simulink model "Eq_1"  (R2014a)
settings: Solver=ode45  StartTime=0.0  StopTime=20  RelTol=1e-3
undefined symbols (not defined in the file or in its folder): dfilt
libraries: dsparch4 x5, dspvision x2, dspsnks4 x1
settings Model: Creator=Misa  LastModifiedBy=Misa

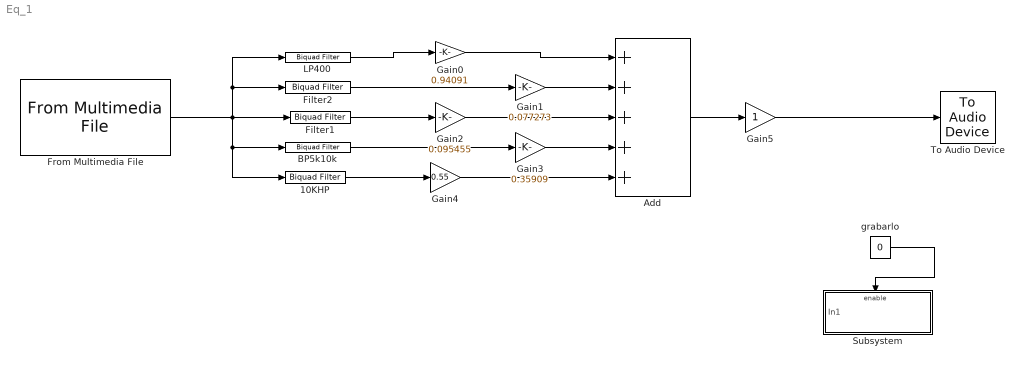
== system Eq_1 ==
  10KHP : dsparch4/Biquad Filter  Tag=BlockMethodSubSystem  IIRFiltStruct=Direct form II  CoeffSource=Specify via dialog  BiQuadCoeffs=[1 -2 1 1 -0.435559960227692333 0.682874457925469414;1 -2 1 1 -0.336863684852461154 0.301541332551575114;1 -2 1 1 -0.287076251600125121 0.109177462139277051;1 -2 1 1 -0.265814507780955722 0.0270283922717663959]  a0Flag=Warning  IC=0  ICnum=0  ICden=0  InputProcessing=Columns as channels (frame based)  denAccumFracLength=30  denProdOutputFracLength=30  secondMemoryFracLength=15  roundingMode=Floor  overflowMode=off  ScaleValues=[0.529608604538290506;0.409601254351009081;0.349063428434850553;0.323210725013180544;1]  optimizeScaleValues=on  ScaleValueMode=Specify via input port (g)  scaleValueFracLength=14  FilterSource=Specify via dialog  dfiltObjectName=dfilt.df2tsos([1 0.3 0.4],[1 0.1 0.2])
  Add : Sum  Inputs=+++++
  BP5k10k : dsparch4/Biquad Filter  Tag=BlockMethodSubSystem  IIRFiltStruct=Direct form II  CoeffSource=Specify via dialog  BiQuadCoeffs=[1 0 -1 1 -0.511936060109229096 0.976812733722258741;1 0 -1 1 -1.5749417552576479 0.98532114132335924;1 0 -1 1 -1.55120780296343908 0.956591366841473167;1 0 -1 1 -0.5026942036248776 0.932090235078945284;1 0 -1 1 -0.496206083464974634 0.889564263737497196;1 0 -1 1 -1.52719342803245395 0.928655042129086672;1 0 -1 1 -1.50288428756205406 0.901464029452747728;1 0 -1 1 -0.492327906370097379 0.849219797568050661;1 0 -1 1 -1.47826174218308015 0.874975513981652409;1 0 -1 1 -0.490928978268946159 0.811036332045524389;1 0 -1 1 -1.45330358333625353 0.849152306076616625;1 0 -1 1 -0.491891608264251601 0.774990857026918945;1 0 -1 1 -1.42798470855204052 0.823963188122787571;1 0 -1 1 -0.495110695998242645 0.741060291658979464;1 0 -1 1 -1.40227778727378527 0.799383332368227784;1 0 -1 1 -0.500493064212129246 0.70922346320206564;1 0 -1 1 -1.37615396097244957 0.775394812461079219;1 0 -1 1 -0.507956573002034784 0.679462697186595799;1 0 -1 1 -1.34958362384959907 0.7519872274617736;1 0 -1 1 -0.517429030514883981 0.651765066895615197;1 0 -1 1 -1.32253733382701011 0.72915845201805296;1 0 -1 1 -0.528846896304387082 0.626123329774780357;1 0 -1 1 -1.29498690690488116 0.706915518856455316;1 0 -1 1 -0.542153758407436959 0.602536556936418166;1 0 -1 1 -1.26690674987356156 0.685275628197983599;1 0 -1 1 -0.557298554215037045 0.581010439505093901;1 0 -1 1 -1.23827548448857305 0.664267261325699687;1 0 -1 1 -0.574233500145569953 0.561557232705398368;1 0 -1 1 -1.20907790720441133 0.643931350446522721;1 0 -1 1 -0.592911698886189553 0.544195276865696909;1 0 -1 1 -1.17930730791784777 0.624322422786211417;1 0 -1 1 -0.613284409671686737 0.528948017042816243;1 0 -1 1 -1.14896813361933203 0.605509593538764546;1 0 -1 1 -0.635298001700298487 0.515842435093875618;1 0 -1 1 -1.11807892346795779 0.587577232772038549;1 0 -1 1 -0.658890668031314686 0.504906817560012877;1 0 -1 1 -1.08667535838030926 0.570625083388540011;1 0 -1 1 -0.683989059197508409 0.496167819434113699;1 0 -1 1 -1.05481316500134237 0.5547675749297305;1 0 -1 1 -0.710505097907362604 0.489646857192791884;1 0 -1 1 -1.02257050610441946 0.540132082055159723;1 0 -1 1 -0.738333343299314659 0.485355978860020243;1 0 -1 1 -0.990049406305708146 0.526855940429187597;1 0 -1 1 -0.767349355898213625 0.483293507046987036;1 0 -1 1 -0.957375744728905631 0.515082173873032012;1 0 -1 1 -0.797409531394399407 0.483439907073740183;1 0 -1 1 -0.924697436908860082 0.504954102663914828;1 0 -1 1 -0.828352780577823244 0.485754450371230106;1 0 -1 1 -0.892180648569675938 0.49660925926267574;1 0 -1 1 -0.860004212382262767 0.490173266415208975]  a0Flag=Warning  IC=0  ICnum=0  ICden=0  InputProcessing=Columns as channels (frame based)  denAccumFracLength=30  denProdOutputFracLength=30  secondMemoryFracLength=15  roundingMode=Floor  overflowMode=off  ScaleValues=[0.318409620604874377;0.318409620604874377;0.312609545517313181;0.312609545517313181;0.307147001457118485;0.307147001457118485;0.302011246073271178;0.302011246073271178;0.29719133618218585;0.29719133618218585;0.292676349944423264;0.292676349944423264;0.288455556702515381;0.288455556702515381;0.284518544849641064;0.284518544849641064;0.280855316314686354;0.280855316314686354;0.277456354711022701;0.277456354711022701;0.274312672892673248;0.274312672892673248;0.271415844571001152;0.271415844571001152;0.268758023742088736;0.268758023742088736;0.266331954933413495;0.266331954933413495;0.264130976673456697;0.264130976673456697;0.262149020097042551;0.262149020097042551;0.260380604202797961;0.260380604202797961;0.258820828960209026;0.258820828960209026;0.257465367207995455;0.257465367207995455;0.2563104560809355;0.2563104560809355;0.255352888538870559;0.255352888538870559;0.254590005441150902;0.254590005441150902;0.254019688505433716;0.254019688505433716;0.253640354405854029;0.253640354405854029;0.253450950197460445;0.253450950197460445;1]  optimizeScaleValues=on  ScaleValueMode=Specify via input port (g)  scaleValueFracLength=14  FilterSource=Specify via dialog  dfiltObjectName=dfilt.df2tsos([1 0.3 0.4],[1 0.1 0.2])
  Filter1 : dsparch4/Biquad Filter  Tag=BlockMethodSubSystem  IIRFiltStruct=Direct form II  CoeffSource=Specify via dialog  BiQuadCoeffs=[1 0 -1 1 -1.49298544457669613 0.972536600913176619;1 0 -1 1 -1.97375600080993996 0.993967196611222681;1 0 -1 1 -1.45434811513615525 0.91992215302516156;1 0 -1 1 -1.96184279045341059 0.981990541850511933;1 0 -1 1 -1.41911007136003064 0.870355402822089896;1 0 -1 1 -1.94995566918991003 0.970098550984774155;1 0 -1 1 -1.38714659148742636 0.823781823951208914;1 0 -1 1 -1.93805449177893774 0.958251256010940966;1 0 -1 1 -1.35833576516020438 0.780137916222685357;1 0 -1 1 -1.92609852985326024 0.946408948977047637;1 0 -1 1 -1.33256154535689264 0.739355628990374436;1 0 -1 1 -1.91404574389860604 0.934531500155876826;1 0 -1 1 -1.3097162226504544 0.701366035921648701;1 0 -1 1 -1.90185198328248095 0.922577639450826381;1 0 -1 1 -1.28970250064079539 0.666102437361354771;1 0 -1 1 -1.88947007254741828 0.910504166064626363;1 0 -1 1 -1.27243533948969301 0.633503055805215709;1 0 -1 1 -1.87684873043618161 0.898265043581852884;1 0 -1 1 -1.86393124983616087 0.885810324816448391;1 0 -1 1 -1.257843732058602 0.603513485803715;1 0 -1 1 -1.85065383861322852 0.8730848306789043;1 0 -1 1 -1.24587258765892894 0.576089065158300606;1 0 -1 1 -1.83694347738664909 0.860026475874825724;1 0 -1 1 -1.23648492746493122 0.551197354350352553;1 0 -1 1 -1.82271508070995703 0.846564084478204637;1 0 -1 1 -1.22966465290023219 0.528820953727261345;1 0 -1 1 -1.8078676351395444 0.832614457983713696;1 0 -1 1 -1.22542025119886655 0.508960967165100642;1 0 -1 1 -1.79227879867224105 0.81807832481258369;1 0 -1 1 -1.22378998315903997 0.491641562843065538;1 0 -1 1 -1.77579711858101463 0.802834570778408141;1 0 -1 1 -1.22484941898211241 0.476916336802188867;1 0 -1 1 -1.75823043384986621 0.786731740493668341;1 0 -1 1 -1.22872277367223726 0.464877654925497041;1 0 -1 1 -1.73932791135376363 0.769575035828907961;1 0 -1 1 -1.23560060637514946 0.455671050426820101;1 0 -1 1 -1.71875093669712986 0.751105539894514784;1 0 -1 1 -1.24576867300432736 0.449518575540772625;1 0 -1 1 -1.69602335791846537 0.730965293920004311;1 0 -1 1 -1.25965744166257498 0.44675892609350043;1 0 -1 1 -1.67044089099015647 0.708635073665359383;1 0 -1 1 -1.27793246767386881 0.447921223551549119;1 0 -1 1 -1.64089382056394095 0.683316374884235245;1 0 -1 1 -1.30167149900252088 0.453871915193899855;1 0 -1 1 -1.60549565687988194 0.653697459997890973;1 0 -1 1 -1.33273565421145501 0.466132696577705508;1 0 -1 1 -1.56082757662151606 0.617543327540308828;1 0 -1 1 -1.3745248473673557 0.487583520094362788;1 0 -1 1 -1.50169156008034421 0.572103291046450191;1 0 -1 1 -1.43222454905332985 0.523165952149703961]  a0Flag=Warning  IC=0  ICnum=0  ICden=0  InputProcessing=Columns as channels (frame based)  denAccumFracLength=30  denProdOutputFracLength=30  secondMemoryFracLength=15  roundingMode=Floor  overflowMode=off  ScaleValues=[0.278758877019711249;0.278758877019711249;0.274235010892847242;0.274235010892847242;0.269949416623545435;0.269949416623545435;0.265898272850538464;0.265898272850538464;0.262077096217103789;0.262077096217103789;0.258480952180539514;0.258480952180539514;0.255104627583005894;0.255104627583005894;0.251942770859943821;0.251942770859943821;0.248990005094146261;0.248990005094146261;0.246241018460196665;0.246241018460196665;0.243690635976798381;0.243690635976798381;0.241333875910699935;0.241333875910699935;0.239165993663095183;0.239165993663095183;0.237182515518972181;0.237182515518972181;0.235379264249513637;0.235379264249513637;0.233752378222758433;0.233752378222758433;0.232298325392703398;0.232298325392703398;0.231013913295886053;0.231013913295886053;0.229896295981367682;0.229896295981367682;0.22894297862939092;0.22894297862939092;0.228151820470753719;0.228151820470753719;0.227521036498562951;0.227521036498562951;0.227049198362456434;0.227049198362456434;0.226735234749033565;0.226735234749033565;0.226578431477934134;0.226578431477934134;1]  optimizeScaleValues=on  ScaleValueMode=Specify via input port (g)  scaleValueFracLength=14  FilterSource=Specify via dialog  dfiltObjectName=dfilt.df2tsos([1 0.3 0.4],[1 0.1 0.2])
  Filter2 : dsparch4/Biquad Filter  Tag=BlockMethodSubSystem  IIRFiltStruct=Direct form II  CoeffSource=Specify via dialog  BiQuadCoeffs=[1 0 -1 1 -1.97596012833583279 0.996179518646341688;1 0 -1 1 -1.99521952400752611 0.99846517290300385;1 0 -1 1 -1.96851859175579458 0.988605912279289512;1 0 -1 1 -1.99214992198348506 0.995399560857654575;1 0 -1 1 -1.96125803930711751 0.981160151075751497;1 0 -1 1 -1.98907166931553103 0.992334325463347544;1 0 -1 1 -1.95422106977926946 0.973886471810042287;1 0 -1 1 -1.98597866945393919 0.989263518702049982;1 0 -1 1 -1.94744837829074435 0.966827443288640342;1 0 -1 1 -1.98286480675969434 0.986181276643283811;1 0 -1 1 -1.94097871703255276 0.960023914274292345;1 0 -1 1 -1.97972395807416657 0.983081835728266129;1 0 -1 1 -1.93484886261720535 0.953514970993309396;1 0 -1 1 -1.97655001571599565 0.979959562422103359;1 0 -1 1 -1.92909358234205852 0.947337896828783887;1 0 -1 1 -1.97333692733050303 0.976809001648254238;1 0 -1 1 -1.92374559023320169 0.941528125333639165;1 0 -1 1 -1.97007875947474664 0.973624950844582338;1 0 -1 1 -1.91883548183865438 0.936119175780525392;1 0 -1 1 -1.96676979377256256 0.970402568314236436;1 0 -1 1 -1.9143916343797609 0.931142558004078413;1 0 -1 1 -1.96340466691835136 0.967137526832149819;1 0 -1 1 -1.91044005607788758 0.926627630350701614;1 0 -1 1 -1.95997856870902565 0.963826226068218328;1 0 -1 1 -1.90700416542813267 0.922601391201267829;1 0 -1 1 -1.95648751545446853 0.960466080136111344;1 0 -1 1 -1.90410447830915297 0.919088181169101071;1 0 -1 1 -1.95292871913744159 0.957055898955894824;1 0 -1 1 -1.90175817912606515 0.916109270630745209;1 0 -1 1 -1.94930107453028612 0.953596383059907016;1 0 -1 1 -1.94560578572206833 0.950090749581463556;1 0 -1 1 -1.89997855308400165 0.913682307011692396;1 0 -1 1 -1.94184714729627905 0.946545499549337643;1 0 -1 1 -1.89877426304988406 0.911820601091401395;1 0 -1 1 -1.93803348047229917 0.942971320297574023;1 0 -1 1 -1.89814846952970728 0.910532244717123462;1 0 -1 1 -1.93417819657065215 0.939384087834612136;1 0 -1 1 -1.89809782037954733 0.909819078328251596;1 0 -1 1 -1.93030091600834464 0.935805889972775251;1 0 -1 1 -1.89861138115352301 0.909675569333436407;1 0 -1 1 -1.9264285118880915 0.932265934195341317;1 0 -1 1 -1.89966963625802165 0.91008772143071337;1 0 -1 1 -1.92259588239113133 0.928801144878157237;1 0 -1 1 -1.90124375605247531 0.911032202623118792;1 0 -1 1 -1.91884620803054484 0.925456215497890478;1 0 -1 1 -1.90329537329813192 0.912475934793618659;1 0 -1 1 -1.91523045088558952 0.922282894079524906;1 0 -1 1 -1.90577711139492223 0.914376398077903385;1 0 -1 1 -1.91180593584687464 0.91933837367792437;1 0 -1 1 -1.90863402403330928 0.916682834119376344]  a0Flag=Warning  IC=0  ICnum=0  ICden=0  InputProcessing=Columns as channels (frame based)  denAccumFracLength=30  denProdOutputFracLength=30  secondMemoryFracLength=15  roundingMode=Floor  overflowMode=off  ScaleValues=[0.0426725602520760042;0.0426725602520760042;0.0425591023286577275;0.0425591023286577275;0.0424472087389355449;0.0424472087389355449;0.0423372884878717506;0.0423372884878717506;0.0422297336523212302;0.0422297336523212302;0.0421249186567085529;0.0421249186567085529;0.0420231997148002578;0.0420231997148002578;0.0419249144219856346;0.0419249144219856346;0.0418303814820186678;0.0418303814820186678;0.0417399005520427413;0.0417399005520427413;0.0416537521898713708;0.0416537521898713708;0.0415721978878865472;0.0415721978878865472;0.0414954801784973223;0.0414954801784973223;0.0414238227968344447;0.0414238227968344447;0.0413574308872055874;0.0413574308872055874;0.0412964912407680282;0.0412964912407680282;0.0412411725528634698;0.0412411725528634698;0.0411916256894802324;0.0411916256894802324;0.0411479839533424943;0.0411479839533424943;0.0411103633411602012;0.0411103633411602012;0.0410788627845955212;0.0410788627845955212;0.0410535643685060389;0.0410535643685060389;0.0410345335210057505;0.0410345335210057505;0.0410218191708421193;0.0410218191708421193;0.041015453868520603;0.041015453868520603;1]  optimizeScaleValues=on  ScaleValueMode=Specify via input port (g)  scaleValueFracLength=14  FilterSource=Specify via dialog  dfiltObjectName=dfilt.df2tsos([1 0.3 0.4],[1 0.1 0.2])
  From Multimedia File : dspvision/From Multimedia File  inputFilename=/Volumes/DANIEL N/DSP 2016/Calvin Harris - Feel so Close (Original Mix).mp3  loop=on  numPlays=inf  outputStreams=Audio only  videoDataType=single  audioDataType=double  inheritSampleTime=on  userDefinedSampleTime=1/30  noAudioOutput=off  isIntensityVideo=off  fourcc=RGB  colorVideoFormat=Separate color signals  outputEOF=off  dataOrg=Column-major  audioFrameSize=1024  computeAudioFrameSize=off  outSamplingMode=Frame based
  Gain0 : Gain  Gain=0.94091
  Gain1 : Gain  Gain=0.077273
  Gain2 : Gain  Gain=0.095455
  Gain3 : Gain  Gain=0.35909
  Gain4 : Gain  Gain=0.55
  Gain5 : Gain
  LP400 : dsparch4/Biquad Filter  Tag=BlockMethodSubSystem  IIRFiltStruct=Direct form II  CoeffSource=Specify via dialog  BiQuadCoeffs=[1 2 1 1 -1.95804317832839403 0.960730291047929508;1 2 1 1 -1.905141444097604 0.907755957333884922]  a0Flag=Warning  IC=0  ICnum=0  ICden=0  InputProcessing=Columns as channels (frame based)  denAccumFracLength=30  denProdOutputFracLength=30  secondMemoryFracLength=15  roundingMode=Floor  overflowMode=off  ScaleValues=[0.000671778179883860131;0.000653628309070184116;1]  optimizeScaleValues=on  ScaleValueMode=Specify via input port (g)  scaleValueFracLength=14  FilterSource=Specify via dialog  dfiltObjectName=dfilt.df2tsos([1 0.3 0.4],[1 0.1 0.2])
  Subsystem : Subsystem
  To Audio Device : dspsnks4/To Audio Device  deviceName=Default  inheritSampleRate=on  sampleRate=44100  deviceDatatype=Determine from input data type  autoBufferSize=on  bufferSize=4096  queueDuration=1  defaultOutputChannelMapping=on  outputChannelMapping=1:2
  grabarlo : Constant  Value=0
  wires:
  LP400/1 -> Gain0/1
  10KHP/1 -> Gain4/1
  Add/1 -> Gain5/1
  BP5k10k/1 -> Gain3/1
  Gain0/1 -> Add/1
  Gain2/1 -> Add/3
  Gain3/1 -> Add/4
  Gain4/1 -> Add/5
  Filter1/1 -> Gain2/1
  From Multimedia File/1 -> LP400/1, Filter2/1, 10KHP/1, BP5k10k/1, Filter1/1
  Filter2/1 -> Gain1/1
  Gain1/1 -> Add/2
  grabarlo/1 -> Subsystem/Enable
  Gain5/1 -> To Audio Device/1

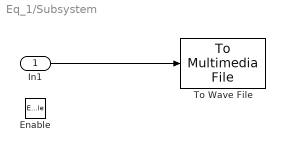
== system Eq_1/Subsystem ==
  In1 : Inport
  Enable : EnablePort
  To Wave File : dspvision/To Multimedia File  outputFilename=/Users/Misa/Desktop/DSP/songecu.wav  streamSelection=Audio only  videoCompressor=None (uncompressed)  audioCompressor=None (uncompressed)  imagePorts=Separate color signals  fileType=WAV  audioDatatype=Determine from input data type  fourcc=RGB  videoQuality=75  mj2000CompFactor=10
  wires:
  In1/1 -> To Wave File/1
